simulink model "FIR_SymmetricStream_Ex1"  (R2023a)
settings: Solver=VariableStepAuto  StartTime=0.0  StopTime=1  RelTol=1e-3
PostLoadFcn:
  | Fs = 100000;  % Sampling Frequency
  | Fpass = 5000;              % Passband Frequency
  | Fstop = 10000;             % Stopband Frequency
  | Dpass = 0.0046051376314;   % Passband Ripple
  | Dstop = 0.00025118864315;  % Stopband Attenuation
  | dens  = 16;                % Density Factor
  | % Calculate the order from the parameters using FIRPMORD.
  | [N, Fo, Ao, W] = firpmord([Fpass, Fstop]/(Fs/2), [1 0], [Dpass, Dstop]);
  | % Calculate the coefficients using the FIRPM function.
  | coeffs = firpm(N, Fo, Ao, W, {dens});
  | AIE_Coeffs = (int16(coeffs(1:32)*2^15));
undefined symbols (not defined in the file): firpmord, None, S, vsva2197, xcvc1902
libraries: dspsrcs4 x1, aieDSP x1, dspmlti4 x1, vmcUtilities x1
settings Model: Creator=sdegala  LastModifiedBy=robg
settings ModelReferenceCC: EnableRefExpFcnMdlSchedulingChecks=on

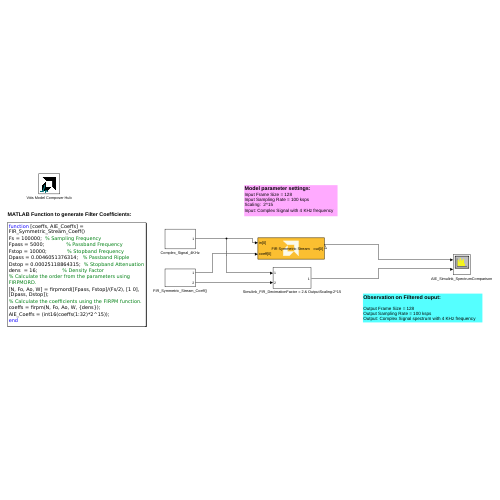
[thumbnail: Simulink's stored preview of the top-level diagram]
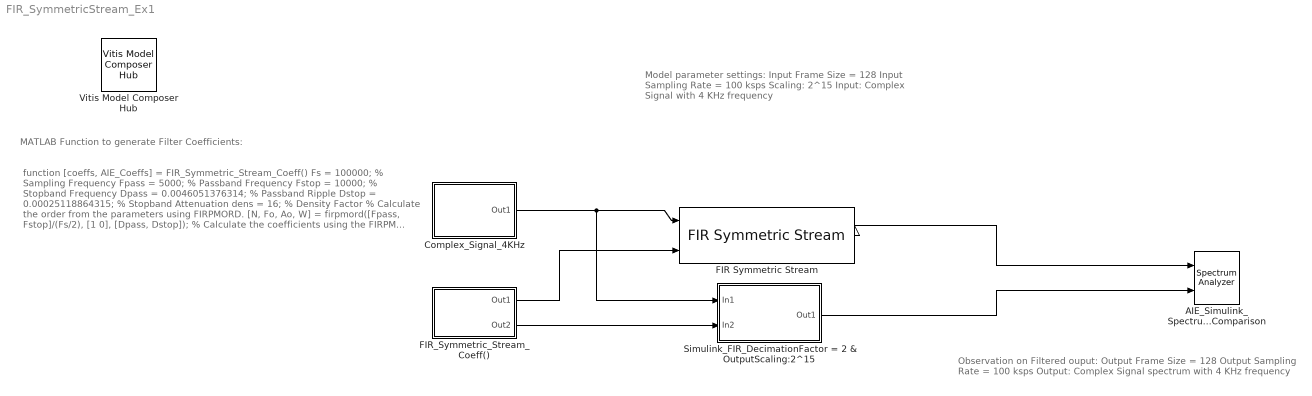
== system FIR_SymmetricStream_Ex1 ==
  note: function [coeffs, AIE_Coeffs] = FIR_Symmetric_Stream_Coeff()
      | Fs = 100000; % Sampling Frequency
      | Fpass = 5000; % Passband Frequency
      | Fstop = 10000; % Stopband Frequency
      | Dpass = 0.0046051376314; % Passband Ripple
      | Dstop = 0.00025118864315; % Stopband Attenuation
      | dens = 16; % Density Factor
      | % Calculate the order from the parameters using FIRPMORD.
      | [N, Fo, Ao, W] = firpmord([Fpass, Fstop]/(Fs/2), [1 0], [Dpass, Dstop]);
      | % Calculate the coefficients using the FIRPM function.
      | coeffs = firpm(N, Fo, Ao, W, {dens});
      | AIE_Coeffs = (int16(coeffs(1:32)*2^15));
      | end
  note: MATLAB Function to generate Filter Coefficients:
  note: Observation on Filtered ouput:
      |
      | Output Frame Size = 128
      | Output Sampling Rate = 100 ksps
      | Output: Complex Signal spectrum with 4 KHz frequency
  note: Model parameter settings:
      | Input Frame Size = 128
      | Input Sampling Rate = 100 ksps
      | Scaling: 2^15
      | Input: Complex Signal with 4 KHz frequency
  AIE_Simulink_SpectrumComparison : SpectrumAnalyzer  NumInputPorts=2  AveragingMethod=Exponential  ShowLegend=on  ChannelNames="[\"\"]"  DefaultConfigurationName=spbscopes.SpectrumAnalyzerBlockCfg
  Complex_Signal_4KHz : Subsystem
  FIR Symmetric Stream : aieDSP/FIR Symmetric Stream  data_type=cint16  coef_type=int16  use_coeff_reload=on  dual_ip=off  num_outputs=off  coeff=[1, zeros(1,15)]  fir_length=64  input_window_size=128  shift_val=15  rnd_mode=Round to positive infinity  sat_mode=0-None  ssr=1  casc_length=1  AIE_VARIANT=1  blockJsonConstraints=[]  blockJsonConstraintsInternal=[]  spec=vmc_stream_fir_sr_sym.json  SerializedMaskParamNames=[]  SerializedMaskParamValues=[]  SerializedMaskParamVisibilities=[]  block_type=FIR Symmetric Stream  SerializedMaskParamDataypes=typename|typename|bool|bool|bool|coef_type|uint|uint|uint|uint|uint|uint|uint|uint  SerializedMaskParamEnumStrArr=0|0|0|0|0|0|0|0|0|Floor,Ceiling,Round to positive infinity,Round to negative infinity,Round symmetrical to infinity,Round symmetrical to zero,Round convergent to even,Round convergent to odd|0-None,1-Asymmetric,3-Symmetric|0|0|0  SerializedMaskParamEnumValArr=0|0|0|0|0|0|0|0|0|0,1,2,3,4,5,6,7|0,1,3|0|0|0  SerializedMaskParamVectorArr=0|0|0|0|0|1|0|0|0|0|0|0|0|0
  FIR_Symmetric_Stream_Coeff() : Subsystem
  Simulink_FIR_DecimationFactor = 2 & OutputScaling:2^15 : Subsystem
  Vitis Model Composer Hub : vmcUtilities/Vitis Model Composer Hub  Tag=genX  CodeGeneration=off  StartColumn=1  NumberOfColumns=1  TargetDirectory=./code  exportDesign=off  analyzeDesign=off  validateDesignOnHw=off  ExportType=AI Engines  IpVendor=xilinx.com  IpLibrary=hls  IpVersion=1.0  IpHWLanguage=Verilog  AieCompilerOptions={}  AieSimulatorOptions={}  CreateTestbench=off  TestbenchStackSize=10  RunRtlSim=off  RunCSim=off  RunAieSim=off  AieSimTimeout=50000  RunAieSimProfiling=off  LaunchVitisAnalyzer=off  PlotOutput=off  RunX86Sim=off  X86SimTimeout=10  GenHwImage=off  GenLibadfXo=off  GenHwValidationCode=off  PlatformType=Not Specified  HwSystemType=Baremetal  HwValidationTarget=hw  ProjDevice=xcvc1902-vsva2197-1LP-e-S  ProjDevicePart=xcvc1902-vsva2197-1LP-e-S  AIEType=AIE  SamplePeriod=-1  ClockFrequency=200  DataPathParallelism=1  xilinxfamily=versalaicore  part=xcvc1902  speed=-1LP-e-S  package=vsva2197  directory=./netlist  testbench=off  incr_netlist=off  synthesis_tool=Vivado  clock_wrapper=Clock Enables  dbl_ovrd=According to Block Masks  dcm_input_clock_period=10  sysclk_period=10  simulink_period=1  eval_field=0  LogFileName=''  NThreads=4
  wires:
  Complex_Signal_4KHz/1(Out1) -> FIR Symmetric Stream/1, Simulink_FIR_DecimationFactor = 2 & OutputScaling:2^15/1(In1)
  FIR Symmetric Stream/1 -> AIE_Simulink_SpectrumComparison/1
  Simulink_FIR_DecimationFactor = 2 & OutputScaling:2^15/1(Out1) -> AIE_Simulink_SpectrumComparison/2
  FIR_Symmetric_Stream_Coeff()/1(Out1) -> FIR Symmetric Stream/2
  FIR_Symmetric_Stream_Coeff()/2(Out2) -> Simulink_FIR_DecimationFactor = 2 & OutputScaling:2^15/2(In2)

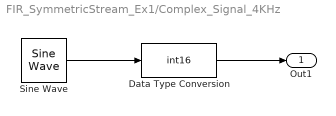
== system FIR_SymmetricStream_Ex1/Complex_Signal_4KHz ==
  Data Type Conversion : DataTypeConversion  OutMin=[-1]  OutMax=[1]  OutDataTypeStr=int16  ConvertRealWorld=Stored Integer (SI)  SaturateOnIntegerOverflow=off  RndMeth=Floor
  Sine Wave : dspsrcs4/Sine Wave  Amplitude=1  Frequency=4e3  Phase=0  SampleMode=Discrete  OutComplex=Complex  CompMethod=Table lookup  TableSize=Speed  SampleTime=1/100e3  SamplesPerFrame=128  ResetState=Restart at time zero  OutputFrames=off  dataType=Fixed-point  wordLen=16  udDataType=sfix(16)  fracBitsMode=User-defined  numFracBits=14  OutDataTypeStr=fixdt(1,16,14)  LastOutDataTypeStr=fixdt(1,16,14)
  Out1 : Outport
  wires:
  Sine Wave/1 -> Data Type Conversion/1
  Data Type Conversion/1 -> Out1/1

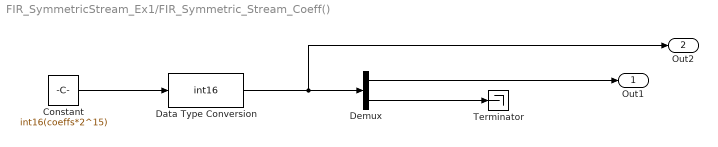
== system FIR_SymmetricStream_Ex1/FIR_Symmetric_Stream_Coeff() ==
  Constant : Constant  Value=int16(coeffs*2^15)
  Data Type Conversion : DataTypeConversion  OutMin=[-1]  OutMax=[1]  OutDataTypeStr=int16  ConvertRealWorld=Stored Integer (SI)  SaturateOnIntegerOverflow=off  RndMeth=Floor
  Demux : Demux  Outputs=2
  Terminator : Terminator
  Out1 : Outport
  Out2 : Outport  Port=2
  wires:
  Demux/2 -> Terminator/1
  Constant/1 -> Data Type Conversion/1
  Demux/1 -> Out1/1
  Data Type Conversion/1 -> Out2/1, Demux/1

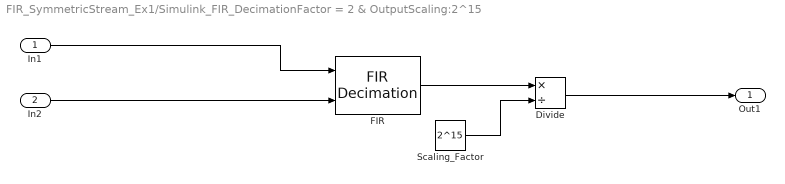
== system FIR_SymmetricStream_Ex1/Simulink_FIR_DecimationFactor = 2 & OutputScaling:2^15 ==
  In1 : Inport
  In2 : Inport  Port=2
  Divide : Product  Inputs=*/  OutDataTypeStr=int16
  FIR : dspmlti4/FIR Decimation  FilterSource=Input port  h=int16(firpm(63, [0;0.1;0.2;1], [1;1;0;0], [1;18.3333831245308], {16})*2^15)  D=1  filtStruct=Direct form  FilterObject=firpmord([5e3, 10e3]/(100e3/2), [1 0], [0.0046051376314, 0.0001995262315])  InputProcessing=Columns as channels (frame based)  framing=Enforce single-rate processing  AllowArbitraryInputLength=off  inputOffset=0  outputBufInitCond=0  roundingMode=Floor  overflowMode=off  firstCoeffDataTypeStr=Inherit: Same word length as input  firstCoeffMin=[]  firstCoeffMax=[]  firstCoeffLastDataTypeStr=Inherit: Same word length as input  prodOutputMode=Binary point scaling  prodOutputWordLength=32  prodOutputFracLength=0  prodOutputDataTypeStr=fixdt(1,32,0)  prodOutputLastDataTypeStr=fixdt(1,32,0)  accumMode=Binary point scaling  accumWordLength=48  accumFracLength=0  accumDataTypeStr=fixdt(1,48,0)  accumLastDataTypeStr=fixdt(1,48,0)  outputDataTypeStr=Inherit: Same as product output  outputMin=[]  outputMax=[]  outputLastDataTypeStr=Inherit: Same as product output
  Scaling_Factor : Constant  Value=2^15  OutDataTypeStr=int32
  Out1 : Outport
  wires:
  Scaling_Factor/1 -> Divide/2
  FIR/1 -> Divide/1
  In1/1 -> FIR/1
  Divide/1 -> Out1/1
  In2/1 -> FIR/2
